simulink model "Simulacion_veocidad"  (R2015b)
settings: Solver=ode4  StartTime=0.0  StopTime=1.98  FixedStep=0.02  RelTol=1e-3
undefined symbols (not defined in the file): de_vel_cont, de_vel_disc, nu_vel_cont, nu_vel_disc
settings Model: Creator=sersanc8  LastModifiedBy=sersanc8

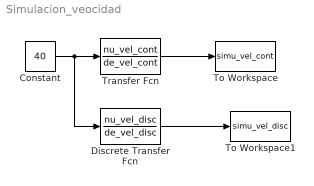
== system Simulacion_veocidad ==
  Constant : Constant  Value=40
  Discrete Transfer Fcn : DiscreteTransferFcn  Numerator=nu_vel_disc  Denominator=de_vel_disc  SampleTime=0.02
  To Workspace : ToWorkspace  VariableName=simu_vel_cont  SampleTime=-1
  To Workspace1 : ToWorkspace  VariableName=simu_vel_disc  SampleTime=-1
  Transfer Fcn : TransferFcn  Numerator=nu_vel_cont  Denominator=de_vel_cont
  wires:
  Constant/1 -> Discrete Transfer Fcn/1, Transfer Fcn/1
  Transfer Fcn/1 -> To Workspace/1
  Discrete Transfer Fcn/1 -> To Workspace1/1
